simulink model "DCM_17"  (R2019b)
settings: Solver=VariableStepAuto  StartTime=0.0  StopTime=20  RelTol=1e-3
undefined symbols (not defined in the file or in its folder): Rarm
libraries: powerlib x23
settings Model: Creator=Sy2  LastModifiedBy=Sy2
settings SolverCC: ZeroCrossAlgorithm=Adaptive
settings DebuggingCC: IgnoredZcDiagnostic=none

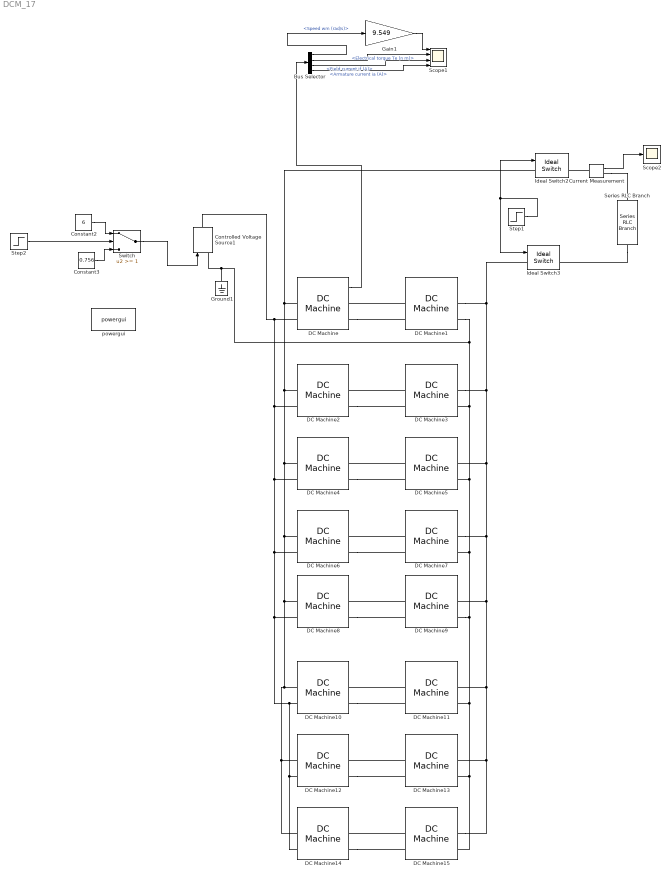
== system DCM_17 ==
  Bus Selector : BusSelector  OutputSignals=Speed wm (rad/s),Electrical torque Te (n m),Field current if (A),Armature current ia (A)
  Constant2 : Constant  Value=6
  Constant3 : Constant  Value=0.756
  Controlled Voltage Source1 : powerlib/Electrical Sources/Controlled Voltage Source  Initialize=on  Source_Type=DC  Amplitude=0  Phase=0  Frequency=0  Measurements=None
      settings: SourceProductName=Simscape Electrical
  Current Measurement : powerlib/Measurements/Current Measurement  PhasorSimulation=off  OutputType=Complex  PSBequivalent=0
      settings: SourceProductName=Simscape Electrical
  DC Machine{,1..15} (16 alike) : powerlib/Machines/DC Machine  PresetModel=No  MechanicalLoad=Torque TL  FieldType=Wound  ShowDetailedParameters=on  MeasurementBus=off  RLa="[Rarm  0.002]"  RLf=[0.0054 0.0125]  Laf=Laf  MachineConstant=Torque constant (N.m/A)  Ke=1.8  Kt=1.8  J=137  Bm=0  Tf=0  w0=initial_speed  Ifinit=0  TsPowergui=0  TsBlock=-1
      settings: SourceProductName=Simscape Electrical
  Gain1 : Gain  Gain=9.549
  Ground1 : powerlib/Elements/Ground  LConnTagsString=a
      settings: SourceProductName=Simscape Electrical
  Ideal Switch2 : powerlib/Power Electronics/Ideal Switch  Ron=0  Lon=0  IC=0  Rs=inf  Cs=0  Measurements=on
      settings: SourceProductName=Simscape Electrical
  Ideal Switch3 : powerlib/Power Electronics/Ideal Switch  Ron=0  Lon=0  IC=0  Rs=inf  Cs=0  Measurements=on
      settings: SourceProductName=Simscape Electrical
  Scope1 : Scope  NumInputPorts=4
  Scope2 : Scope
  Series RLC Branch : powerlib/Elements/Series RLC Branch  LConnTagsString=__new0  RConnTagsString=__new0  BranchType=RL  Resistance=0.09  Inductance=0.0245  SetiL0=off  InitialCurrent=0  Capacitance=1e-6  Setx0=off  InitialVoltage=0  Measurements=None
      settings: SourceProductName=Simscape Electrical
  Step1 : Step  Time=13  SampleTime=0  VectorParams1D=off
  Step2 : Step  Time=0  SampleTime=0  VectorParams1D=off  ZeroCross=off
  Switch : Switch  Threshold=1  ZeroCross=off
  powergui : powerlib/powergui  Priority=1  SimulationMode=Continuous  SampleTime=50e-6  frequency=60  Iterations=50  frequencyindice=0  Pbase=100e6  ErrMax=1e-4  UnitsV=kV  UnitsW=MW  buscounter=0  FunctionMessages=off  echomessages=off  EnableUseOfTLC=off  CurrentSourceSwitches=off  DisableSnubberDevices=off  DisableRonSwitches=off  DisableVfSwitches=off  DisplayEquations=off  AutomaticDiscreteSolvers=off  SolverType=Tustin/Backward Euler (TBE)  Interpol=off  ExternalGateDelay=off  methode=off  Ts=100  x0status=blocks  SPID=on  SwTol=0  HookPort=off  NonlinearTolerance=1e-4  nMaxIteration=100  ContinueOnMaxIteration=off  RestoreLinks=warning  ResistiveCurrentMeasurement=off  Frange=[0:2:500]  Ylog=off  Xlog=on  ShowGrid=off  save=off  variable=ZData  structure=0  ZoomFFT=off  StartTime=0.0  cycles=1  DisplayStyle=1  fundamental=60  FreqAxis=off  MaxFrequency=1000  frequencyindicesteady=1  RmsSteady=1  display=off
      settings: SourceProductName=Simscape Electrical
  wires:
  DC Machine/1 -> Bus Selector/1
  Bus Selector/1 -> Gain1/1  "<Speed wm (rad/s)>"
  Bus Selector/2 -> Scope1/2  "<Electrical torque Te (n m)>"
  Bus Selector/3 -> Scope1/3  "<Field current if (A)>"
  Bus Selector/4 -> Scope1/4  "<Armature current ia (A)>"
  Gain1/1 -> Scope1/1
  Step1/1 -> Ideal Switch3/1, Ideal Switch2/1
  Switch/1 -> Controlled Voltage Source1/1
  Constant3/1 -> Switch/3
  Step2/1 -> Switch/2
  Constant2/1 -> Switch/1
  Current Measurement/1 -> Scope2/1
  connections:
  Series RLC Branch/RConn1 -- Ideal Switch3/RConn1
  Current Measurement/LConn1 -- Ideal Switch2/RConn1
  Current Measurement/RConn1 -- Series RLC Branch/LConn1
  DC Machine1/LConn1 -- DC Machine/RConn1
  DC Machine/RConn2 -- DC Machine1/LConn2
  DC Machine8/LConn2 -- DC Machine4/LConn2 -- DC Machine2/LConn2 -- DC Machine/LConn2 -- Controlled Voltage Source1/RConn1 -- DC Machine6/LConn2 -- DC Machine14/LConn2 -- DC Machine12/LConn2 -- DC Machine10/LConn2
  DC Machine15/RConn2 -- DC Machine13/RConn2 -- DC Machine9/RConn2 -- DC Machine5/RConn2 -- Controlled Voltage Source1/LConn1 -- Ground1/LConn1 -- DC Machine1/RConn2 -- DC Machine3/RConn2 -- DC Machine7/RConn2 -- DC Machine11/RConn2
  DC Machine2/RConn2 -- DC Machine3/LConn2
  DC Machine3/LConn1 -- DC Machine2/RConn1
  DC Machine4/RConn2 -- DC Machine5/LConn2
  DC Machine5/LConn1 -- DC Machine4/RConn1
  DC Machine15/RConn1 -- DC Machine11/RConn1 -- DC Machine5/RConn1 -- DC Machine1/RConn1 -- Ideal Switch3/LConn1 -- DC Machine3/RConn1 -- DC Machine7/RConn1 -- DC Machine9/RConn1 -- DC Machine13/RConn1
  DC Machine6/RConn2 -- DC Machine7/LConn2
  DC Machine7/LConn1 -- DC Machine6/RConn1
  DC Machine12/RConn2 -- DC Machine13/LConn2
  DC Machine13/LConn1 -- DC Machine12/RConn1
  DC Machine14/RConn2 -- DC Machine15/LConn2
  DC Machine8/RConn2 -- DC Machine9/LConn2
  DC Machine10/RConn2 -- DC Machine11/LConn2
  DC Machine11/LConn1 -- DC Machine10/RConn1
  DC Machine9/LConn1 -- DC Machine8/RConn1
  DC Machine15/LConn1 -- DC Machine14/RConn1
  DC Machine6/LConn1 -- Ideal Switch2/LConn1 -- DC Machine/LConn1 -- DC Machine2/LConn1 -- DC Machine4/LConn1 -- DC Machine14/LConn1 -- DC Machine12/LConn1 -- DC Machine10/LConn1 -- DC Machine8/LConn1
